simulink model "TemplateMatchingContinuous"  (R2020a)
settings: Solver=VariableStepAuto  StartTime=0  StopTime=180  RelTol=1e-3
values from neighbouring files (symbols this model uses):
  buffer_rec = length(template)    [run_TemplateMatchingCentered.m]    (also in run_TemplateMatchingContinuous.m = length(template1))
  fs = 30000    [run_TemplateMatchingCentered.m]    (also in run_TemplateMatchingContinuous.m)
  refractory = 10^-3    (= 0.001)    [run_TemplateMatchingCentered.m]    (also in run_TemplateMatchingContinuous.m)
  score = [3000]    [run_TemplateMatchingCentered.m]    (also in run_TemplateMatchingContinuous.m = [3000:25:3600])
  template1 = double(mean_waveform{1, 1}(:,str2num(ch(3:end))))'    [run_TemplateMatchingContinuous.m]
  template2 = double(mean_waveform{1, 2}(:,str2num(ch(3:end))))'    [run_TemplateMatchingContinuous.m]
  template3 = double(mean_waveform{1, 3}(:,str2num(ch(3:end))))'    [run_TemplateMatchingContinuous.m]
libraries: simulink x4, dspswit3 x3, dspfdesign x2, hdlsllib x1
settings Model: SimulationMode=rapid-accelerator  Creator=sbuccelli  LastModifiedBy=diflo

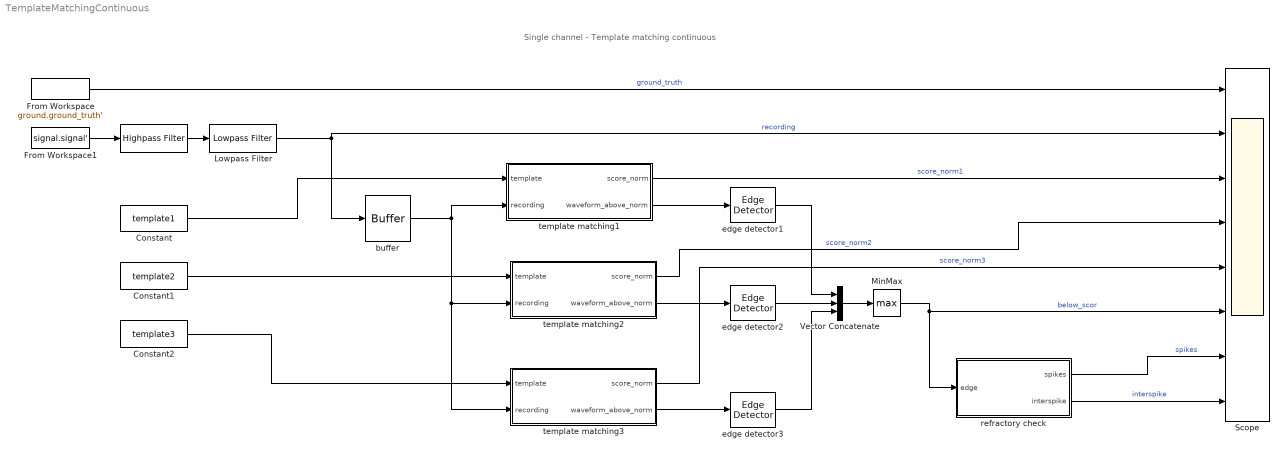
== system TemplateMatchingContinuous ==
  note: Single channel - Template matching continuous
  " " : dspfdesign/Highpass Filter  FilterType=IIR  DesignForMinimumOrder=on  FilterOrder=50  StopbandFrequency=1  PassbandFrequency=300  StopbandAttenuation=80  PassbandRipple=0.1  InheritSampleRate=off  SampleRate=fs  SimulateUsing=Interpreted execution  roundingMode=Floor  coeffsDataTypeStr=fixdt(1,16)
  Constant : Constant  Value=template1
  Constant1 : Constant  Value=template2
  Constant2 : Constant  Value=template3
  From Workspace : FromWorkspace  VariableName=ground.ground_truth'  SampleTime=1/fs
  From Workspace1 : FromWorkspace  VariableName=signal.signal'  SampleTime=1/fs
  Lowpass Filter : dspfdesign/Lowpass Filter  FilterType=IIR  DesignForMinimumOrder=on  FilterOrder=3  PassbandFrequency=3500  StopbandFrequency=8500  PassbandRipple=0.1  StopbandAttenuation=80  InheritSampleRate=off  SampleRate=fs  SimulateUsing=Interpreted execution  roundingMode=Floor  coeffsDataTypeStr=fixdt(1,16)
  MinMax : MinMax  Function=max
  Scope : Scope  NumInputPorts=8
  Vector Concatenate : Concatenate  NumInputs=3
  buffer : Buffer  N=buffer_rec  V=buffer_overlap  OutputFrames=off
  edge detector1 : dspswit3/Edge Detector  InputProcessing=Columns as channels (frame based)
      settings: SourceProductBaseCode=DS
  edge detector2 : dspswit3/Edge Detector  InputProcessing=Columns as channels (frame based)
      settings: SourceProductBaseCode=DS
  edge detector3 : dspswit3/Edge Detector  InputProcessing=Columns as channels (frame based)
      settings: SourceProductBaseCode=DS
  refractory check : Subsystem
  template matching1 : Subsystem
  template matching2 : Subsystem
  template matching3 : Subsystem
  wires:
  Constant/1 -> template matching1/1(template)
  Lowpass Filter/1 -> Scope/2, buffer/1  "recording"
  buffer/1 -> template matching1/2(recording), template matching3/2(recording), template matching2/2(recording)
  " "/1 -> Lowpass Filter/1
  From Workspace1/1 -> " "/1
  Constant1/1 -> template matching2/1(template)
  Constant2/1 -> template matching3/1(template)
  template matching1/2(waveform_above_norm) -> edge detector1/1
  template matching2/2(waveform_above_norm) -> edge detector2/1
  edge detector3/1 -> Vector Concatenate/3
  template matching3/2(waveform_above_norm) -> edge detector3/1
  edge detector1/1 -> Vector Concatenate/1
  edge detector2/1 -> Vector Concatenate/2
  Vector Concatenate/1 -> MinMax/1
  MinMax/1 -> Scope/6, refractory check/1("  edge")  "below_scor"
  refractory check/2(interspike) -> Scope/8  "interspike"
  refractory check/1(" spikes") -> Scope/7  "spikes"
  From Workspace/1 -> Scope/1  "ground_truth"
  template matching1/1(score_norm) -> Scope/3  "score_norm1"
  template matching2/1(score_norm) -> Scope/4  "score_norm2"
  template matching3/1(score_norm) -> Scope/5  "score_norm3"

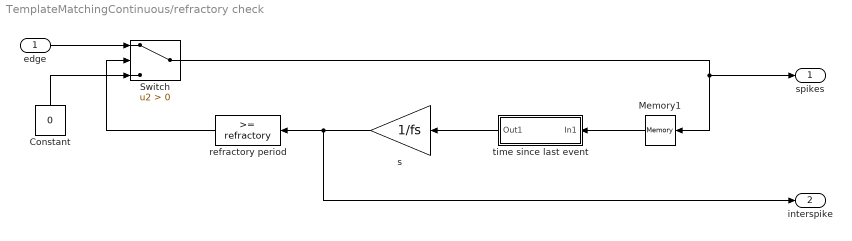
== system TemplateMatchingContinuous/refractory check ==
  "  edge" : Inport
  Constant : Constant  Value=0
  Memory1 : Memory  InheritSampleTime=on
  Switch : Switch  Criteria=u2 > Threshold
  refractory period : simulink/Logic and Bit Operations/Compare To Constant  relop=>=  const=refractory  OutDataTypeStr=boolean
  s : Gain  Gain=1/fs  ParamDataTypeStr=double
  time since last event : Subsystem
  " spikes" : Outport
  interspike : Outport  Port=2
  wires:
  "  edge"/1 -> Switch/1
  Memory1/1 -> time since last event/1(In1)
  time since last event/1(Out1) -> s/1
  Constant/1 -> Switch/3
  s/1 -> refractory period/1, interspike/1
  Switch/1 -> " spikes"/1, Memory1/1
  refractory period/1 -> Switch/2

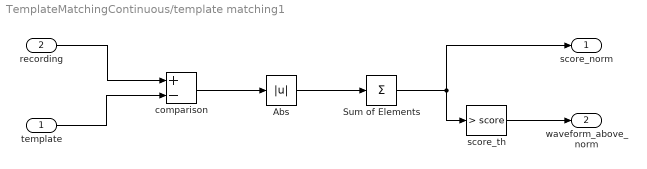
== system TemplateMatchingContinuous/template matching1 ==
  template : Inport
  recording : Inport  Port=2
  Abs : Abs
  Sum of Elements : Sum  Inputs=+
  comparison : Sum  Inputs=+-
  score_th : simulink/Logic and Bit Operations/Compare To Constant  relop=>  const=score  OutDataTypeStr=boolean
  score_norm : Outport
  waveform_above_norm : Outport  Port=2
  wires:
  Abs/1 -> Sum of Elements/1
  comparison/1 -> Abs/1
  Sum of Elements/1 -> score_th/1, score_norm/1
  recording/1 -> comparison/1
  score_th/1 -> waveform_above_norm/1
  template/1 -> comparison/2

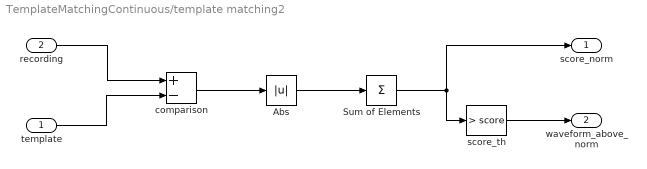
== system TemplateMatchingContinuous/template matching2 ==
  template : Inport
  recording : Inport  Port=2
  Abs : Abs
  Sum of Elements : Sum  Inputs=+
  comparison : Sum  Inputs=+-
  score_th : simulink/Logic and Bit Operations/Compare To Constant  relop=>  const=score  OutDataTypeStr=boolean
  score_norm : Outport
  waveform_above_norm : Outport  Port=2
  wires:
  Abs/1 -> Sum of Elements/1
  comparison/1 -> Abs/1
  Sum of Elements/1 -> score_th/1, score_norm/1
  recording/1 -> comparison/1
  score_th/1 -> waveform_above_norm/1
  template/1 -> comparison/2

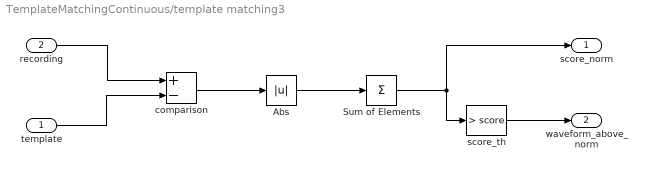
== system TemplateMatchingContinuous/template matching3 ==
  template : Inport
  recording : Inport  Port=2
  Abs : Abs
  Sum of Elements : Sum  Inputs=+
  comparison : Sum  Inputs=+-
  score_th : simulink/Logic and Bit Operations/Compare To Constant  relop=>  const=score  OutDataTypeStr=boolean
  score_norm : Outport
  waveform_above_norm : Outport  Port=2
  wires:
  Abs/1 -> Sum of Elements/1
  comparison/1 -> Abs/1
  Sum of Elements/1 -> score_th/1, score_norm/1
  recording/1 -> comparison/1
  score_th/1 -> waveform_above_norm/1
  template/1 -> comparison/2

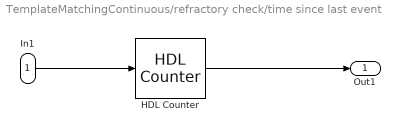
== system TemplateMatchingContinuous/refractory check/time since last event ==
  In1 : Inport
  HDL Counter : hdlsllib/Sources/HDL Counter  CountType=Free running  CountInit=1  CountStep=1  CountMax=25  CountFromType=Initial value  CountFrom=1  CountResetPort=on  CountLoadPort=off  CountEnbPort=off  CountDirPort=off  CountDataType=Unsigned  CountWordLen=32  CountFracLen=0  CountSampTime=1
  Out1 : Outport
  wires:
  In1/1 -> HDL Counter/1
  HDL Counter/1 -> Out1/1
